simulink model "Gravidade (1)"  (R2017a)
settings: Solver=VariableStepAuto  StartTime=0.0  StopTime=252  RelTol=1e-3
libraries: simulink x1
settings Model: Creator=13199959938  LastModifiedBy=13199959938

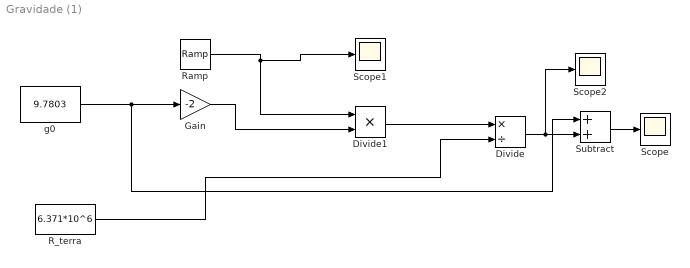
== system Gravidade (1) ==
  Divide : Product  Inputs=*/
  Divide1 : Product  Inputs=**
  Gain : Gain  Gain=-2
  R_terra : Constant  Value=6.371*10^6
  Ramp : simulink/Sources/Ramp  slope=25.67  start=0  X0=0
  Scope : Scope
  Scope1 : Scope
  Scope2 : Scope
  Subtract : Sum
  g0 : Constant  Value=9.7803
  wires:
  g0/1 -> Subtract/1, Gain/1
  Gain/1 -> Divide1/2
  R_terra/1 -> Divide/2
  Ramp/1 -> Scope1/1, Divide1/1
  Divide1/1 -> Divide/1
  Divide/1 -> Scope2/1, Subtract/2
  Subtract/1 -> Scope/1
